simulink model "Motor_Position"  (R2020b)
settings: Solver=VariableStepAuto  StartTime=0.0  StopTime=10.0  RelTol=1e-3
model workspace (MAT data in the model file):
  J = 3.2284e-06
  K = 0.0274
  L = 2.75e-06
  R = 4
  b = 3.5077e-06
settings Model: Creator=sai  LastModifiedBy=sai
settings DataIOCC: SaveOutput=off  SaveTime=off

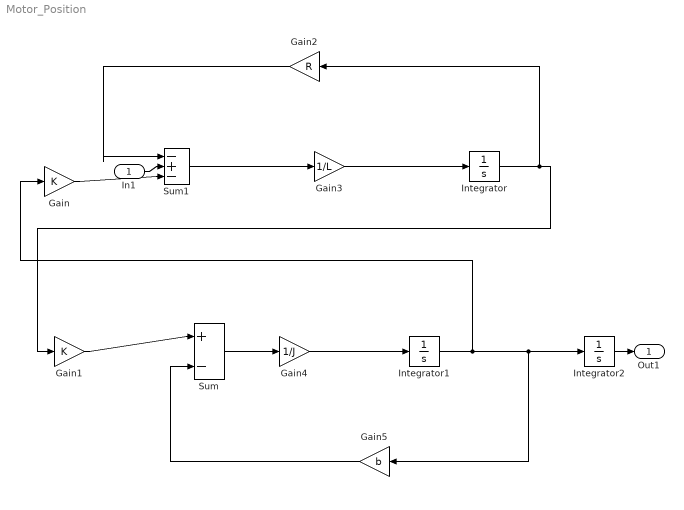
== system Motor_Position ==
  In1 : Inport  OutDataTypeStr=double  PortDimensions=1  SampleTime=0
  Gain : Gain  Gain=K
  Gain1 : Gain  Gain=K
  Gain2 : Gain  Gain=R
  Gain3 : Gain  Gain=1/L
  Gain4 : Gain  Gain=1/J
  Gain5 : Gain  Gain=b
  Integrator : Integrator
  Integrator1 : Integrator
  Integrator2 : Integrator
  Sum : Sum  Inputs=|+-
  Sum1 : Sum  Inputs=|-+-
  Out1 : Outport  OutDataTypeStr=double  PortDimensions=1  SampleTime=0
  wires:
  Gain1/1 -> Sum/1
  Gain/1 -> Sum1/3
  Sum1/1 -> Gain3/1
  Gain5/1 -> Sum/2
  Integrator2/1 -> Out1/1
  Integrator1/1 -> Integrator2/1, Gain5/1, Gain/1
  Gain3/1 -> Integrator/1
  Gain4/1 -> Integrator1/1
  Gain2/1 -> Sum1/1
  Integrator/1 -> Gain1/1, Gain2/1
  Sum/1 -> Gain4/1
  In1/1 -> Sum1/2
